simulink model "test"  (R2021a)
settings: Solver=ode4  StartTime=0.0  StopTime=t_final  FixedStep=dt  RelTol=1e-3
values from neighbouring files (symbols this model uses):
  e_IC = e_IC_1(i)    [HW3_c.m]    (also in HW3_e.m = 40.6)
  K = 60    [HW3_a.m]    (also in HW3_b.m = 100; HW3_c.m; HW3_d.m = 1; HW3_e.m = 100)
undefined symbols (not defined in the file or in its folder): A, B, C, D
settings Model: Creator=CF  LastModifiedBy=msi-PC
settings SolverCC: AlgebraicLoopSolver=TrustRegion
settings DataIOCC: ReturnWorkspaceOutputs=off
settings DebuggingCC: SFMachineParentedDataDiag=warning  ArithmeticOperatorsInVariantConditions=warning
settings SFSimCC: SimUseLocalCustomCode=off  CustomCodeUndefinedFunction=UseInterfaceOnly
settings RTWCC: RTWUseLocalCustomCode=off

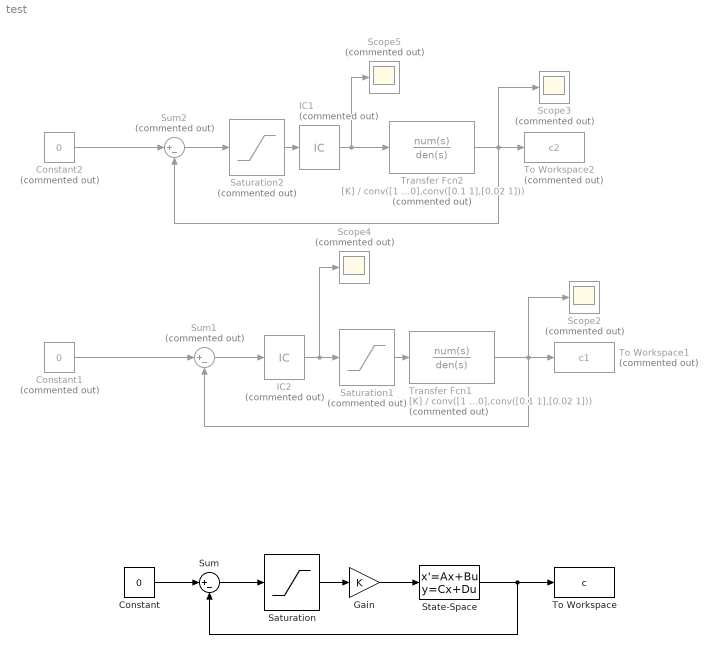
== system test ==
  Constant : Constant  Value=0
  Constant1 : Constant  Commented=on  Value=0
  Constant2 : Constant  Commented=on  Value=0
  Gain : Gain  Gain=K
  IC1 : InitialCondition  Commented=on  Value=e_IC
  IC2 : InitialCondition  Commented=on  Value=e_IC
  Saturation : Saturate  UpperLimit=20  LowerLimit=-20
  Saturation1 : Saturate  Commented=on  UpperLimit=20  LowerLimit=-20
  Saturation2 : Saturate  Commented=on  UpperLimit=20  LowerLimit=-20
  Scope{2..5} (4 alike) : Scope  Commented=on
  State-Space : StateSpace  A=A  B=B  C=C  D=D  InitialCondition=[0 0 -e_IC/500]
  Sum : Sum  Inputs=|+-
  Sum1 : Sum  Commented=on  Inputs=|+-
  Sum2 : Sum  Commented=on  Inputs=|+-
  To Workspace : ToWorkspace  VariableName=c  SampleTime=-1
  To Workspace1 : ToWorkspace  Commented=on  VariableName=c1  SampleTime=-1
  To Workspace2 : ToWorkspace  Commented=on  VariableName=c2  SampleTime=-1
  Transfer Fcn1 : TransferFcn  Commented=on  Numerator=[K]  Denominator=conv([1 0],conv([0.1 1],[0.02 1]))
  Transfer Fcn2 : TransferFcn  Commented=on  Numerator=[K]  Denominator=conv([1 0],conv([0.1 1],[0.02 1]))
  wires:
  Saturation/1 -> Gain/1
  State-Space/1 -> To Workspace/1, Sum/2
  Constant1/1 -> Sum1/1
  Transfer Fcn1/1 -> Scope2/1, Sum1/2, To Workspace1/1
  Saturation1/1 -> Transfer Fcn1/1
  Sum1/1 -> IC2/1
  IC2/1 -> Scope4/1, Saturation1/1
  Constant2/1 -> Sum2/1
  Transfer Fcn2/1 -> Scope3/1, Sum2/2, To Workspace2/1
  Sum2/1 -> Saturation2/1
  IC1/1 -> Scope5/1, Transfer Fcn2/1
  Saturation2/1 -> IC1/1
  Sum/1 -> Saturation/1
  Constant/1 -> Sum/1
  Gain/1 -> State-Space/1
